simulink model "feedback"  (R2018b)
settings: Solver=VariableStepAuto  StartTime=0.0  StopTime=5.0  RelTol=1e-3
values from neighbouring files (symbols this model uses):
  A = [0 1 0 0 ... (first row only)    [nonlinearsim.m]    (also in stability.m = [0,1,0,0; 0,0,(-m*g)/((j/R^2)+m),0; 0,0,0,1; 0,0,0,0])
  B = [0; 0; 0; 1]    [nonlinearsim.m]    (also in stability.m = [0;0;0;1])
  C = [1 0 0 0]    [nonlinearsim.m]    (also in stability.m = [1,0,0,0])
  K = [ -17.1874  -22.0571   71.0000   14.0000]    [nonlinearsim.m]    (also in stability.m = acker(A,B,p))
  N = -17.1874    [nonlinearsim.m]    (also in stability.m = inv(g))
settings Model: Creator=hasti  LastModifiedBy=hasti

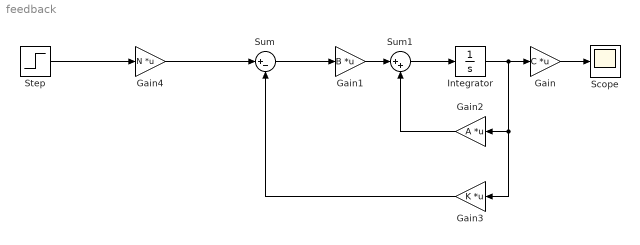
== system feedback ==
  Gain : Gain  Gain=C  Multiplication=Matrix(K*u)
  Gain1 : Gain  Gain=B  Multiplication=Matrix(K*u)
  Gain2 : Gain  Gain=A  Multiplication=Matrix(K*u)
  Gain3 : Gain  Gain=K  Multiplication=Matrix(K*u)
  Gain4 : Gain  Gain=N  Multiplication=Matrix(K*u)
  Integrator : Integrator  InitialCondition=-5
  Scope : Scope
  Step : Step  SampleTime=0
  Sum : Sum  Inputs=|+-
  Sum1 : Sum  Inputs=|++
  wires:
  Gain1/1 -> Sum1/1
  Sum/1 -> Gain1/1
  Sum1/1 -> Integrator/1
  Integrator/1 -> Gain3/1, Gain2/1, Gain/1
  Gain2/1 -> Sum1/2
  Gain3/1 -> Sum/2
  Gain/1 -> Scope/1
  Gain4/1 -> Sum/1
  Step/1 -> Gain4/1
